simulink model "three_phase_ac_regulator"  (Simulink 6.1)
settings: Solver=ode23tb  StartTime=0.0  StopTime=0.15  MaxStep=1e-4  RelTol=1e-3  AbsTol=.01
libraries: powerlib x9
settings Model: LastModifiedBy=ThinkPad
settings DebuggingCC: SolverPrmCheckMsg=warning

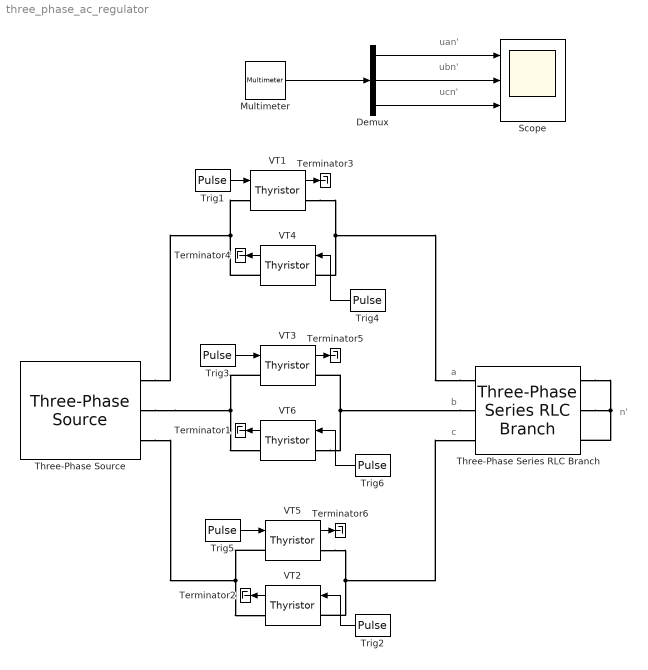
== system three_phase_ac_regulator ==
  note: n'
  note: uan'
  note: ubn'
  note: ucn'
  note: a
  note: b
  note: c
  Demux : Demux  Outputs=3
  Multimeter : powerlib/Measurements/Multimeter  PhasorSimulation=off  OutputType=Complex  sel=[1 2 3]  L=3  Gain=[1 1 1]  yselected={'Ub1: Three-Phase Series RLC Branch','Ub2: Three-Phase Series RLC Branch','Ub3: Three-Phase Series RLC Branch'};  PSBOutputType=1  PSBequivalent=0  AxesSetting=[0,0.1,-100,100]  Display=0  SavedBlockNames=-11
  Scope : Scope  NumInputPorts=3
      settings: TimeRange=0.05  YMin=-100~-100~-100  YMax=100~100~100  SampleTime=1e-4
  Terminator{1..6} (6 alike) : Terminator
  Three-Phase Series RLC Branch : powerlib/Elements/Three-Phase Series RLC Branch  PhysicalDomain=powersysdomain  SubClassName=unknown  LeftPortType=p1  RightPortType=p1  LConnTagsString=A|B|C  RConnTagsString=A|B|C  Resistance=10  Inductance=0  Capacitance=inf  Measurements=Branch voltages
  Three-Phase Source : powerlib/Electrical Sources/Three-Phase Source  Voltage=100  PhaseAngle=0  Frequency=50  InternalConnection=Yg  SpecifyImpedance=off  Resistance=0.1  Inductance=1e-4  ShortCircuitLevel=100e6  BaseVoltage=25e3  XRratio=7
  Trig1 : DiscretePulseGenerator  PulseType=Time based  Amplitude=10  Period=0.02  PulseWidth=20  PhaseDelay=0.005
  Trig2 : DiscretePulseGenerator  Orientation=left  PulseType=Time based  Amplitude=10  Period=0.02  PulseWidth=20  PhaseDelay=0.00833
  Trig3 : DiscretePulseGenerator  PulseType=Time based  Amplitude=10  Period=0.02  PulseWidth=20  PhaseDelay=0.01167
  Trig4 : DiscretePulseGenerator  Orientation=left  PulseType=Time based  Amplitude=10  Period=0.02  PulseWidth=20  PhaseDelay=0.015
  Trig5 : DiscretePulseGenerator  PulseType=Time based  Amplitude=10  Period=0.02  PulseWidth=20  PhaseDelay=0.01833
  Trig6 : DiscretePulseGenerator  Orientation=left  PulseType=Time based  Amplitude=10  Period=0.02  PulseWidth=20  PhaseDelay=0.00167
  VT1 : powerlib/Power Electronics/Thyristor  Ron=0.01  Lon=0  Vf=0.8  IC=0  Rs=1000  Cs=100e-9  Measurements=on
  VT2 : powerlib/Power Electronics/Thyristor  Orientation=left  Ron=0.01  Lon=0  Vf=0.8  IC=0  Rs=1000  Cs=100e-9  Measurements=on
  VT3 : powerlib/Power Electronics/Thyristor  Ron=0.01  Lon=0  Vf=0.8  IC=0  Rs=1000  Cs=100e-9  Measurements=on
  VT4 : powerlib/Power Electronics/Thyristor  Orientation=left  Ron=0.01  Lon=0  Vf=0.8  IC=0  Rs=1000  Cs=100e-9  Measurements=on
  VT5 : powerlib/Power Electronics/Thyristor  Ron=0.01  Lon=0  Vf=0.8  IC=0  Rs=1000  Cs=100e-9  Measurements=on
  VT6 : powerlib/Power Electronics/Thyristor  Orientation=left  Ron=0.01  Lon=0  Vf=0.8  IC=0  Rs=1000  Cs=100e-9  Measurements=on
  wires:
  Trig1/1 -> VT1/1
  Trig4/1 -> VT4/1
  Multimeter/1 -> Demux/1
  Demux/1 -> Scope/1
  Demux/2 -> Scope/2
  Demux/3 -> Scope/3
  Trig3/1 -> VT3/1
  Trig6/1 -> VT6/1
  Trig5/1 -> VT5/1
  Trig2/1 -> VT2/1
  VT5/1 -> Terminator6/1
  VT3/1 -> Terminator5/1
  VT1/1 -> Terminator3/1
  VT2/1 -> Terminator2/1
  VT6/1 -> Terminator1/1
  VT4/1 -> Terminator4/1
  connections:
  Three-Phase Series RLC Branch/LConn1 -- VT1/RConn1 -- VT4/LConn1
  VT4/RConn1 -- VT1/LConn1 -- Three-Phase Source/RConn1
  VT3/LConn1 -- VT6/RConn1 -- Three-Phase Source/RConn2
  Three-Phase Series RLC Branch/LConn2 -- VT6/LConn1 -- VT3/RConn1
  VT5/RConn1 -- VT2/LConn1 -- Three-Phase Series RLC Branch/LConn3
  VT5/LConn1 -- VT2/RConn1 -- Three-Phase Source/RConn3
  Three-Phase Series RLC Branch/RConn1 -- Three-Phase Series RLC Branch/RConn3 -- Three-Phase Series RLC Branch/RConn2
